simulink model "exp_5"  (R2013b)
settings: Solver=ode45  StartTime=0.0  StopTime=10.0  RelTol=1e-3
libraries: simulink x1
settings Model: Creator=lenovo  LastModifiedBy=lenovo

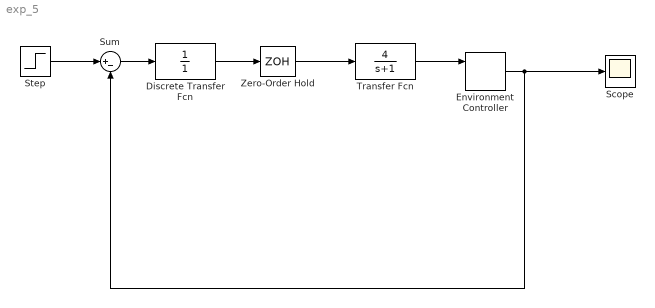
== system exp_5 ==
  Discrete Transfer Fcn : DiscreteTransferFcn  Denominator=[1]
  Environment Controller : simulink/Signal Routing/Environment Controller
  Scope : Scope
  Step : Step  SampleTime=0
  Sum : Sum  Inputs=|+-
  Transfer Fcn : TransferFcn  Numerator=4  Denominator=[1 1]
  Zero-Order Hold : ZeroOrderHold
  wires:
  Step/1 -> Sum/1
  Sum/1 -> Discrete Transfer Fcn/1
  Discrete Transfer Fcn/1 -> Zero-Order Hold/1
  Zero-Order Hold/1 -> Transfer Fcn/1
  Transfer Fcn/1 -> Environment Controller/1
  Environment Controller/1 -> Sum/2, Scope/1
